simulink library "control_gen"  (R2018b)
settings: Solver=VariableStepAuto  StartTime=0.0  StopTime=10.0  RelTol=1e-3
undefined symbols (not defined in the file): P
libraries: aerolibutil x2
settings Model: Creator=colem  LastModifiedBy=colem

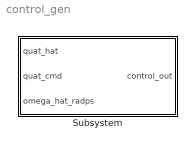
== system control_gen ==
  Subsystem : Subsystem

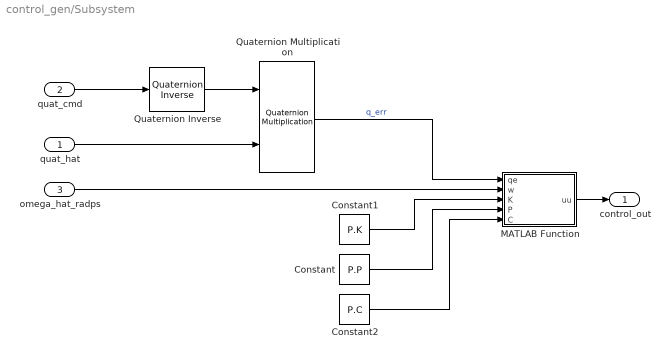
== system control_gen/Subsystem ==
  quat_hat : Inport
  quat_cmd : Inport  Port=2
  omega_hat_radps : Inport  Port=3
  Constant : Constant  Value=P.P
  Constant1 : Constant  Value=P.K
  Constant2 : Constant  Value=P.C
  MATLAB Function : MATLAB Function  TreatAsAtomicUnit=on
  Quaternion Inverse : aerolibutil/Quaternion Inverse
      settings: SourceProductName=Aerospace Blockset
  Quaternion Multiplication : aerolibutil/Quaternion Multiplication
  control_out : Outport
  wires:
  Quaternion Inverse/1 -> Quaternion Multiplication/1
  quat_hat/1 -> Quaternion Multiplication/2
  Quaternion Multiplication/1 -> MATLAB Function/1(qe)  "q_err"
  MATLAB Function/1(uu) -> control_out/1
  omega_hat_radps/1 -> MATLAB Function/2(w)
  quat_cmd/1 -> Quaternion Inverse/1
  Constant/1 -> MATLAB Function/4(P)
  Constant1/1 -> MATLAB Function/3(K)
  Constant2/1 -> MATLAB Function/5(C)

== matlab function control_gen/Subsystem/MATLAB Function ==
  data: qe input; uu output; w input; K input; P input; C input
function uu = fcn(qe, w, K, P, C)
uu = zeros(3,1);

uu = -saturation_norm(K*saturation_1(P*qe(2:4)) + C*w);
end
